simulink model "scheme3"  (R2014a)
settings: Solver=ode45  StartTime=0.0  StopTime=10.0  RelTol=1e-3
settings Model: Creator=Valentin  LastModifiedBy=Valentin

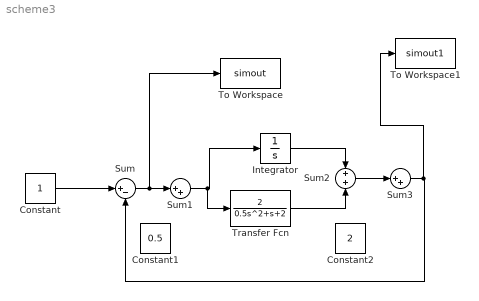
== system scheme3 ==
  Constant : Constant
  Constant1 : Constant  Value=0.5
  Constant2 : Constant  Value=2
  Integrator : Integrator
  Sum : Sum  Inputs=|+-
  Sum1 : Sum  Inputs=|++
  Sum2 : Sum
  Sum3 : Sum  Inputs=|++
  To Workspace : ToWorkspace  VariableName=simout  SaveFormat=Timeseries  SampleTime=-1
  To Workspace1 : ToWorkspace  VariableName=simout1  SaveFormat=Timeseries  SampleTime=-1
  Transfer Fcn : TransferFcn  Numerator=[2]  Denominator=[0.5 1 2]
  wires:
  Sum1/1 -> Transfer Fcn/1, Integrator/1
  Sum/1 -> To Workspace/1, Sum1/1
  Integrator/1 -> Sum2/1
  Transfer Fcn/1 -> Sum2/2
  Sum2/1 -> Sum3/1
  Sum3/1 -> To Workspace1/1, Sum/2
  Constant/1 -> Sum/1
